simulink model "Wind_Turbine_Flexible_Blades"  (Simulink 7.9)
settings: Solver=ode15s  StartTime=0.0  StopTime=10  RelTol=1e-5
PreLoadFcn:
  | load ss_cantilever_pva.mat
  | warning('off','Simulink:SL_SaveWithParameterizedLinks_Warning');
PostLoadFcn:
  | loadMass = 20; %kg
InitFcn:
  | cantilever1=cantilever_aluminum;
  | load1.mass = 20 ; %kg
  | load1.inertia = eye(3) ; % assume point mass
  | load2=load1;
  | load2.angle = 35 * pi / 180;
undefined symbols (not defined in the file or in its folder): Flex_Blade
libraries: mblibv1 x21, Flex_Cantilever_Lib x3
Description:
  | Copyright 2011 MathWorks, Inc.
settings Model: Creator=smiller  LastModifiedBy=smiller
settings OptimizationCC: InitFltsAndDblsToZero=on
settings DebuggingCC: AlgebraicLoopMsg=none  ArtificialAlgebraicLoopMsg=none  SolverPrmCheckMsg=none  FcnCallInpInsideContextMsg=Use local settings  StrictBusMsg=Warning
settings GRTTargetCC: CombineOutputUpdateFcns=off  GRTInterface=on
settings SimMechanicsCC: VisSampleTime=0.1  AnimationDelay=0  LastVizWinPosition=[597 463 560 420]  CamPosition=[0.113022;0.0247231;-11.6929;]  CamTarget=[0.113022;0.0247231;-0;]  CamUpVector=[0;1;0;]  CamHeight=0.95142  VisBackgroundColor=[0.9;0.9;0.95;]  DefaultBodyColor=[1;0;0;]
settings ConfigurationSet: Description=SimMechanics 2G

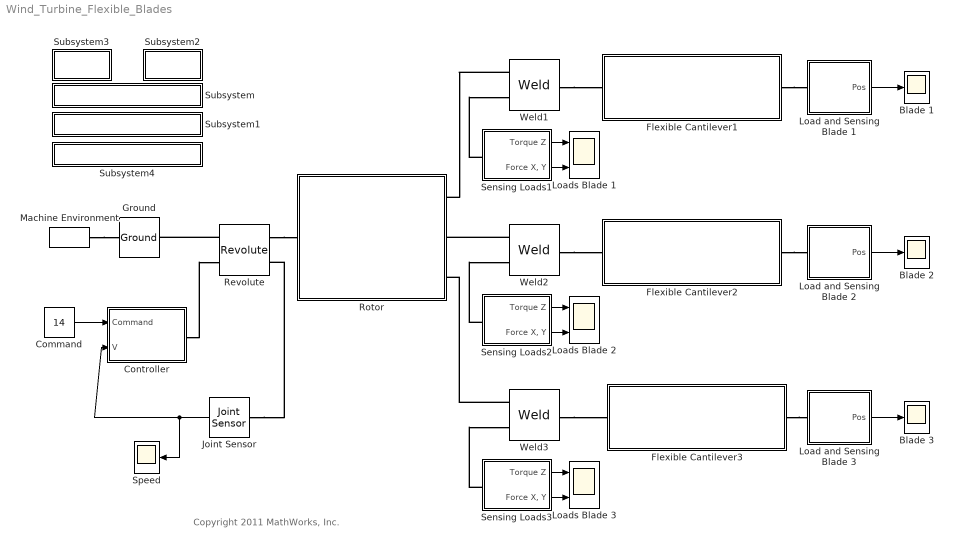
== system Wind_Turbine_Flexible_Blades ==
  note: Copyright 2011 MathWorks, Inc.
  Blade 1 : Scope
      settings: TimeRange=10  YMin=-0.6  YMax=0.6  SaveName=Flex_Beam_Tip_DATA1
  Blade 2 : Scope
      settings: TimeRange=10  YMin=-0.6  YMax=0.6  SaveName=Flex_Beam_Tip_DATA
  Blade 3 : Scope
      settings: TimeRange=10  YMin=-0.6  YMax=0.6  SaveName=Flex_Beam_Tip_DATA2
  Command : Constant  Value=14
  Controller : Subsystem
  Flexible Cantilever1 : Subsystem  BlockChoice=Lumped Parameter
      link override FEA Modes/Deflection due to flexibility/SIZED_INPUT_PORT: PortDimensions=3
      link override FEA Modes/Reaction Force on base (flexible body)/MSB_SIGNAL_BLOCK: Value=[0 0 0]
      link override Lumped Parameter/Beam1/Joint Sensor/MSB_SIGNAL_BLOCK: Value=0
      settings: AttributesFormatString=%<BlockChoice>  TemplateBlock=Flex_Cantilever_Lib/Flexible Cantilever  MemberBlocks=FEA Modes,Lumped Parameter
  Flexible Cantilever2 : Subsystem  BlockChoice=Lumped Parameter
      link override FEA Modes/Deflection due to flexibility/SIZED_INPUT_PORT: PortDimensions=3
      link override FEA Modes/Reaction Force on base (flexible body)/MSB_SIGNAL_BLOCK: Value=[0 0 0]
      link override Lumped Parameter/Beam1/Joint Sensor/MSB_SIGNAL_BLOCK: Value=0
      settings: AttributesFormatString=%<BlockChoice>  TemplateBlock=Flex_Cantilever_Lib/Flexible Cantilever  MemberBlocks=FEA Modes,Lumped Parameter
  Flexible Cantilever3 : Subsystem  BlockChoice=Lumped Parameter
      link override FEA Modes/Deflection due to flexibility/SIZED_INPUT_PORT: PortDimensions=3
      link override FEA Modes/Reaction Force on base (flexible body)/MSB_SIGNAL_BLOCK: Value=[0 0 0]
      link override Lumped Parameter/Beam1/Joint Sensor/MSB_SIGNAL_BLOCK: Value=0
      settings: AttributesFormatString=%<BlockChoice>  TemplateBlock=Flex_Cantilever_Lib/Flexible Cantilever  MemberBlocks=FEA Modes,Lumped Parameter
  Ground : mblibv1/Bodies/Ground  UpdateFromCAD=off  LeftPortType=env  RightPortType=workingframe  PhysicalDomain=Mechanical  DialogClass=GroundBlock  CoordPosition=[0 0 0]  CoordPositionUnits=m  StateVectorMgrId=-1  MachineId=[0 0]  ShowEnvPort=on
  Joint Sensor : mblibv1/Sensors &  Actuators/Joint Sensor  UpdateFromCAD=off  PhysicalDomain=Mechanical  PortType=blob  Muxed=off  Pose=off  Angle=off  AngleUnits=deg  ArcVelocity=on  ArcVelocityUnits=rpm  ArcAcceleration=off  ArcAccelerationUnits=deg/s^2  CoordPosition=on  CoordPositionUnits=m  Velocity=off  VelocityUnits=m/s  Acceleration=off  AccelerationUnits=m/s^2  Quaternion=on  QuaternionDT=off  QuaternionDDT=off  QuaternionUnits=off  OutputVector=[1]  ActiveIO=on  Width=1  DialogClass=MechanicalSensorBlock  Primitive=R1  Force=off  ForceUnits=N  Torque=off  TorqueUnits=N*m  ReferenceFrame=Absolute (World)  ReactionSensedSide=Base  ReactionReferenceFrame=Absolute (World)  ReactionForce=off  ReactionForceUnits=N  ReactionMoment=off  ReactionMomentUnits=N*m
  Load and Sensing Blade 1 : Subsystem
  Load and Sensing Blade 2 : Subsystem
  Load and Sensing Blade 3 : Subsystem
  Loads Blade 1 : Scope  NumInputPorts=2
      settings: TimeRange=10  YMin=-200~-400  YMax=200~200  SaveName=Flexible_Blade1_Load_DATA
  Loads Blade 2 : Scope  NumInputPorts=2
      settings: YMin=-400~-500  YMax=200~200
  Loads Blade 3 : Scope  NumInputPorts=2
      settings: YMin=-400~-500  YMax=200~200  SaveName=ScopeData3
  Machine Environment : mblibv1/Bodies/Machine Environment  Tag=Factory ground  PortType=env  PhysicalDomain=Mechanical  DialogTemplateClass=MECH.MachineEnvironment  SyncWhenCopied=off  Gravity=[0 -9.81 0]  GravityUnits=m/s^2  GravityAsSignal=off  Dimensionality=Auto-detect  AnalysisType=Forward dynamics  LinearAssemblyTolerance=1e-3  LinearAssemblyToleranceUnits=m  AngularAssemblyTolerance=1e-3  AngularAssemblyToleranceUnits=rad  ConstraintSolverType=Stabilizing  ConstraintRelTolerance=1e-4  ConstraintAbsTolerance=1e-4  UseRobustSingularityHandling=off  RedundancyAnalysisToleranceType=Automatically select tolerance  RedundancyAnalysisTolerance=1e-14  StatePerturbationType=Fixed  PerturbationSize=1e-5  VisualizeMachine=off  BodyVisualizationType=Use model default body geometries  BodyColorSelMode=Use model default  DefaultBodyColor=[1 0 0]
  Revolute : mblibv1/Joints/Revolute  LConnTagsString=__newl0|SA1  RConnTagsString=__newr0|SA1  UpdateFromCAD=off  NumSAPorts=2  CutJoint=off  MarkAsCut=off  Primitives=prismatic  PrimitiveProps=R1$World$[0 0 1]$revolute  DialogClass=JointBlock  R1Axis=[0 0 1]
  Rotor : Subsystem  mask(Disk){radius=0.325/8, width=0.06, mass=0.35, axis_pop=Z, x_angle=90, z_angle=0}
      mask prompts: radius "Radius (m)"; width "Length (m)"; mass "Mass (kg)"; axis_pop "Axis of Symmetry in ADJ Ref Frame"
      mask help: Represents a user-defined rigid body in the form of a cylinder. This dialog sets the mass, radius, length, and axis of symmetry. Axis of symmetry is defined by choosing the X, Y, or Z axis of the coordinate system attached to the ADJ port, which is parameterized using the ADJOINING option. The location of this body is parameterized to the coordinate system attached to the ADJ port.
      mask init:
      | if(strcmp(get_param(gcb,'axis_pop'),'X'))
      |     set_param(gcb,'x_angle','0');
      |     set_param(gcb,'z_angle','90');
      | elseif(strcmp(get_param(gcb,'axis_pop'),'Y'))
      |     set_param(gcb,'x_angle','0');
      |     set_param(gcb,'z_angle','0');
      | elseif(strcmp(get_param(gcb,'axis_pop'),'Z'))
      |     set_param(gcb,'x_angle','90');
      |     set_param(gcb,'z_angle','0');
      | end
      mask Help: Creates a cylindrical body
      mask StyleString: edit,edit,edit,popup(X|Y|Z),edit,edit
  Sensing Loads1 : Subsystem
  Sensing Loads2 : Subsystem
  Sensing Loads3 : Subsystem
  Speed : Scope
      settings: TimeRange=10  YMin=0  YMax=15  SaveName=Flexible_Blade_Rotor_Speed_DATA
  Subsystem : Subsystem
      settings: OpenFcn=Change_Flex_Body_To_FEA_Approach;
      mask Display: disp('Use FEA Modes')
  Subsystem1 : Subsystem
      settings: OpenFcn=Change_Flex_Body_To_Lumped_Parameter;
      mask Display: disp('Use Lumped Parameter')
  Subsystem2 : Subsystem
      settings: OpenFcn=|
      | Temp_ENVHa= get_param(find_system(gcs,'LookUnderMasks','all','FollowLinks','on','ClassName','Environment'),'handle');
      | 
      | set_param(Temp_ENVHa{1},'VisualizeMachine','off');
      | 
      | set_param(gcs,'VisDuringSimulation','off')
      | set_param(gcs,'VisOnUpdateDiagram','off')
      mask Display: disp('Vis Off')
  Subsystem3 : Subsystem
      settings: OpenFcn=|
      | Temp_ENVHa= get_param(find_system(gcs,'LookUnderMasks','all','FollowLinks','on','ClassName','Environment'),'handle');
      | 
      | set_param(Temp_ENVHa{1},'VisualizeMachine','on');
      | clear Temp_ENVHa;
      | set_param(gcs,'VisDuringSimulation','on')
      | set_param(gcs,'VisOnUpdateDiagram','on')
      mask Display: disp('Vis On')
  Subsystem4 : Subsystem
      settings: OpenFcn=Flexible_Blades_Slide_Prep;
      mask Display: disp('Show Methods')
  Weld1 : mblibv1/Joints/Weld  LConnTagsString=__newl0|SA1  RConnTagsString=__newr0  UpdateFromCAD=off  NumSAPorts=1  CutJoint=off  MarkAsCut=off  Primitives=weld  PrimitiveProps=W$World$[0 0 0]$weld  DialogClass=JointBlock  WAxis=[0 0 0]
  Weld2 : mblibv1/Joints/Weld  LConnTagsString=__newl0|SA1  RConnTagsString=__newr0  UpdateFromCAD=off  NumSAPorts=1  CutJoint=off  MarkAsCut=off  Primitives=weld  PrimitiveProps=W$World$[0 0 0]$weld  DialogClass=JointBlock  WAxis=[0 0 0]
  Weld3 : mblibv1/Joints/Weld  LConnTagsString=__newl0|SA1  RConnTagsString=__newr0  UpdateFromCAD=off  NumSAPorts=1  CutJoint=off  MarkAsCut=off  Primitives=weld  PrimitiveProps=W$World$[0 0 0]$weld  DialogClass=JointBlock  WAxis=[0 0 0]
  wires:
  Load and Sensing Blade 3/1(Pos) -> Blade 3/1
  Sensing Loads3/1(Torque Z) -> Loads Blade 3/1
  Load and Sensing Blade 1/1(Pos) -> Blade 1/1
  Sensing Loads1/1(Torque Z) -> Loads Blade 1/1
  Sensing Loads1/2("Force X, Y") -> Loads Blade 1/2
  Sensing Loads2/1(Torque Z) -> Loads Blade 2/1
  Sensing Loads2/2("Force X, Y") -> Loads Blade 2/2
  Joint Sensor/1 -> Controller/2(V), Speed/1
  Command/1 -> Controller/1(Command)
  Load and Sensing Blade 2/1(Pos) -> Blade 2/1
  Sensing Loads3/2("Force X, Y") -> Loads Blade 3/2
  connections:
  Sensing Loads1/LConn1 -- Weld1/LConn2
  Controller/RConn1 -- Revolute/LConn2
  Joint Sensor/LConn1 -- Revolute/RConn2
  Weld2/RConn1 -- Flexible Cantilever2/LConn1
  Weld2/LConn1 -- Rotor/RConn2
  Flexible Cantilever2/RConn1 -- Load and Sensing Blade 2/LConn1
  Sensing Loads2/LConn1 -- Weld2/LConn2
  Weld1/RConn1 -- Flexible Cantilever1/LConn1
  Revolute/LConn1 -- Ground/RConn1
  Flexible Cantilever1/RConn1 -- Load and Sensing Blade 1/LConn1
  Weld1/LConn1 -- Rotor/RConn1
  Revolute/RConn1 -- Rotor/LConn1
  Weld3/LConn1 -- Rotor/RConn3
  Sensing Loads3/LConn1 -- Weld3/LConn2
  Flexible Cantilever3/RConn1 -- Load and Sensing Blade 3/LConn1
  Weld3/RConn1 -- Flexible Cantilever3/LConn1
  Machine Environment/RConn1 -- Ground/LConn1

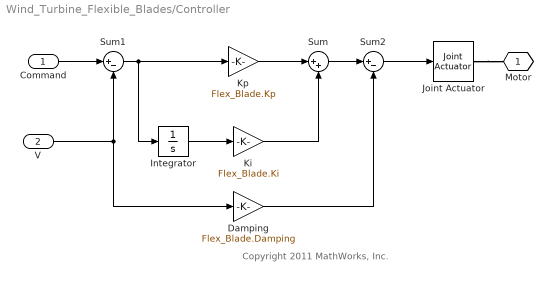
== system Wind_Turbine_Flexible_Blades/Controller ==
  note: Copyright 2011 MathWorks, Inc.
  Command : Inport
  V : Inport  Port=2
  Damping : Gain  Gain=Flex_Blade.Damping
  Integrator : Integrator
  Joint Actuator : mblibv1/Sensors &  Actuators/Joint Actuator  UpdateFromCAD=off  PhysicalDomain=Mechanical  PortType=blob  ActuationStyle=Force  AngleUnits=deg  ArcVelocityUnits=deg/s  ArcAccelerationUnits=deg/s^2  CoordPositionUnits=m  VelocityUnits=m/s  AccelerationUnits=m/s^2  ForceUnits=N  TorqueUnits=N*m  ActiveIO=on  Width=1  DialogClass=MechanicalActuatorBlock  Primitive=R1  ReferenceFrame=Absolute (World)
  Ki : Gain  Gain=Flex_Blade.Ki
  Kp : Gain  Gain=Flex_Blade.Kp
  Sum : Sum  Inputs=|++
  Sum1 : Sum  Inputs=|+-
  Sum2 : Sum  Inputs=|+-
  Motor : PMIOPort  Tag=PMCPort  Port=1  Side=Right
  wires:
  Sum1/1 -> Integrator/1, Kp/1
  Integrator/1 -> Ki/1
  Kp/1 -> Sum/1
  Ki/1 -> Sum/2
  Command/1 -> Sum1/1
  V/1 -> Sum1/2, Damping/1
  Sum/1 -> Sum2/1
  Sum2/1 -> Joint Actuator/1
  Damping/1 -> Sum2/2
  connections:
  Joint Actuator/RConn1 -- Motor/RConn1

== system Wind_Turbine_Flexible_Blades/Flexible Cantilever1 ==
  Lumped Parameter : Flex_Cantilever_Lib/Lumped Parameter  SystemSampleTime=-1
  Base : PMIOPort  Port=1  Side=Left
  Tip : PMIOPort  Port=2  Side=Right
  connections:
  Lumped Parameter/LConn1 -- Base/RConn1
  Lumped Parameter/RConn1 -- Tip/RConn1

== system Wind_Turbine_Flexible_Blades/Flexible Cantilever2 ==
  Lumped Parameter : Flex_Cantilever_Lib/Lumped Parameter  SystemSampleTime=-1
  Base : PMIOPort  Port=1  Side=Left
  Tip : PMIOPort  Port=2  Side=Right
  connections:
  Lumped Parameter/LConn1 -- Base/RConn1
  Lumped Parameter/RConn1 -- Tip/RConn1

== system Wind_Turbine_Flexible_Blades/Flexible Cantilever3 ==
  Lumped Parameter : Flex_Cantilever_Lib/Lumped Parameter  SystemSampleTime=-1
  Base : PMIOPort  Port=1  Side=Left
  Tip : PMIOPort  Port=2  Side=Right
  connections:
  Lumped Parameter/LConn1 -- Base/RConn1
  Lumped Parameter/RConn1 -- Tip/RConn1

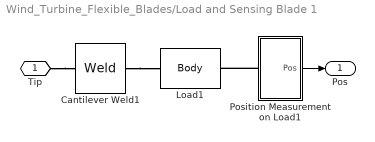
== system Wind_Turbine_Flexible_Blades/Load and Sensing Blade 1 ==
  Cantilever Weld1 : mblibv1/Joints/Weld  LConnTagsString=__newl0  RConnTagsString=__newr0  UpdateFromCAD=off  NumSAPorts=0  CutJoint=off  MarkAsCut=off  Primitives=weld  PrimitiveProps=W$WORLD$[0 0 0]$weld  DialogClass=JointBlock  WAxis=[0 0 0]
  Load1 : mblibv1/Bodies/Body  LConnTagsString=CS1  RConnTagsString=CS2  UpdateFromCAD=off  DialogClass=MechanicalBodyBlock  Mass=loadMass  MassUnits=kg  InertiaUnits=kg*m^2  Inertia=eye(3)  Shape=Cylinder  ShapeDims=[1 1]  ShapeUnits=m  ShapeUse=false  Density=1  DensityUnits=kg/m^3  DensityUse=false  GraphicsMode=1  BodyColorSelMode=MACHINE_DEFAULT  BodyColor=[0.5 0.5 0.5]  AttachedToCS=1  CG=Left$CG$[0 0 0]$CS1$CS1$m$[0 0 0]$Euler X-Y-Z$deg$CS1$false$none  WorkingFrames=Left$CS1$[0 0 0]$Adjoining$Adjoining$m$[0 0 0]$Euler X-Y-Z$deg$Adjoining$true$none#Right$CS2$[0 0 0]$CG$CG$m$[0 0 0]$Euler X-Y-Z$deg$CS1$true$none  CGPos=[0 0 0]  CGRot=[0 0 0]  CS0Pos=[]  CS0Rot=[]  CS1Pos=[0 0 0]  CS1Rot=[0 0 0]  CS2Pos=[0 0 0]  CS2Rot=[0 0 0]  CS3Pos=[]  CS3Rot=[]  CS4Pos=[]  CS4Rot=[]  CS5Pos=[]  CS5Rot=[]  CS6Pos=[]  CS6Rot=[]  CS7Pos=[]  CS7Rot=[]  CS8Pos=[]  CS8Rot=[]  CS9Pos=[]  CS9Rot=[]  CS10Pos=[]  CS10Rot=[]  CS11Pos=[]  CS11Rot=[]  CS12Pos=[]  CS12Rot=[]  CS13Pos=[]  CS13Rot=[]  CS14Pos=[]  CS14Rot=[]  CS15Pos=[]  CS15Rot=[]  CS16Pos=[]  CS16Rot=[]  CS17Pos=[]  CS17Rot=[]  CS18Pos=[]  CS18Rot=[]  CS19Pos=[]  CS19Rot=[]  CS20Pos=[]  CS20Rot=[]
  Position Measurement on Load1 : Subsystem
  Tip : PMIOPort  Port=1  Side=Left
  Pos : Outport
  wires:
  Position Measurement on Load1/1(Pos) -> Pos/1
  connections:
  Cantilever Weld1/LConn1 -- Load1/LConn1
  Position Measurement on Load1/LConn1 -- Load1/RConn1
  Tip/RConn1 -- Cantilever Weld1/RConn1

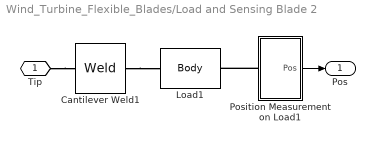
== system Wind_Turbine_Flexible_Blades/Load and Sensing Blade 2 ==
  Cantilever Weld1 : mblibv1/Joints/Weld  LConnTagsString=__newl0  RConnTagsString=__newr0  UpdateFromCAD=off  NumSAPorts=0  CutJoint=off  MarkAsCut=off  Primitives=weld  PrimitiveProps=W$WORLD$[0 0 0]$weld  DialogClass=JointBlock  WAxis=[0 0 0]
  Load1 : mblibv1/Bodies/Body  LConnTagsString=CS1  RConnTagsString=CS2  UpdateFromCAD=off  DialogClass=MechanicalBodyBlock  Mass=loadMass  MassUnits=kg  InertiaUnits=kg*m^2  Inertia=eye(3)  Shape=Cylinder  ShapeDims=[1 1]  ShapeUnits=m  ShapeUse=false  Density=1  DensityUnits=kg/m^3  DensityUse=false  GraphicsMode=1  BodyColorSelMode=MACHINE_DEFAULT  BodyColor=[0.5 0.5 0.5]  AttachedToCS=1  CG=Left$CG$[0 0 0]$CS1$CS1$m$[0 0 0]$Euler X-Y-Z$deg$CS1$false$none  WorkingFrames=Left$CS1$[0 0 0]$Adjoining$Adjoining$m$[0 0 0]$Euler X-Y-Z$deg$Adjoining$true$none#Right$CS2$[0 0 0]$CG$CG$m$[0 0 0]$Euler X-Y-Z$deg$CS1$true$none  CGPos=[0 0 0]  CGRot=[0 0 0]  CS0Pos=[]  CS0Rot=[]  CS1Pos=[0 0 0]  CS1Rot=[0 0 0]  CS2Pos=[0 0 0]  CS2Rot=[0 0 0]  CS3Pos=[]  CS3Rot=[]  CS4Pos=[]  CS4Rot=[]  CS5Pos=[]  CS5Rot=[]  CS6Pos=[]  CS6Rot=[]  CS7Pos=[]  CS7Rot=[]  CS8Pos=[]  CS8Rot=[]  CS9Pos=[]  CS9Rot=[]  CS10Pos=[]  CS10Rot=[]  CS11Pos=[]  CS11Rot=[]  CS12Pos=[]  CS12Rot=[]  CS13Pos=[]  CS13Rot=[]  CS14Pos=[]  CS14Rot=[]  CS15Pos=[]  CS15Rot=[]  CS16Pos=[]  CS16Rot=[]  CS17Pos=[]  CS17Rot=[]  CS18Pos=[]  CS18Rot=[]  CS19Pos=[]  CS19Rot=[]  CS20Pos=[]  CS20Rot=[]
  Position Measurement on Load1 : Subsystem
  Tip : PMIOPort  Port=1  Side=Left
  Pos : Outport
  wires:
  Position Measurement on Load1/1(Pos) -> Pos/1
  connections:
  Tip/RConn1 -- Cantilever Weld1/RConn1
  Position Measurement on Load1/LConn1 -- Load1/RConn1
  Cantilever Weld1/LConn1 -- Load1/LConn1

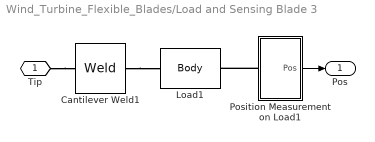
== system Wind_Turbine_Flexible_Blades/Load and Sensing Blade 3 ==
  Cantilever Weld1 : mblibv1/Joints/Weld  LConnTagsString=__newl0  RConnTagsString=__newr0  UpdateFromCAD=off  NumSAPorts=0  CutJoint=off  MarkAsCut=off  Primitives=weld  PrimitiveProps=W$WORLD$[0 0 0]$weld  DialogClass=JointBlock  WAxis=[0 0 0]
  Load1 : mblibv1/Bodies/Body  LConnTagsString=CS1  RConnTagsString=CS2  UpdateFromCAD=off  DialogClass=MechanicalBodyBlock  Mass=loadMass  MassUnits=kg  InertiaUnits=kg*m^2  Inertia=eye(3)  Shape=Cylinder  ShapeDims=[1 1]  ShapeUnits=m  ShapeUse=false  Density=1  DensityUnits=kg/m^3  DensityUse=false  GraphicsMode=1  BodyColorSelMode=MACHINE_DEFAULT  BodyColor=[0.5 0.5 0.5]  AttachedToCS=1  CG=Left$CG$[0 0 0]$CS1$CS1$m$[0 0 0]$Euler X-Y-Z$deg$CS1$false$none  WorkingFrames=Left$CS1$[0 0 0]$Adjoining$Adjoining$m$[0 0 0]$Euler X-Y-Z$deg$Adjoining$true$none#Right$CS2$[0 0 0]$CG$CG$m$[0 0 0]$Euler X-Y-Z$deg$CS1$true$none  CGPos=[0 0 0]  CGRot=[0 0 0]  CS0Pos=[]  CS0Rot=[]  CS1Pos=[0 0 0]  CS1Rot=[0 0 0]  CS2Pos=[0 0 0]  CS2Rot=[0 0 0]  CS3Pos=[]  CS3Rot=[]  CS4Pos=[]  CS4Rot=[]  CS5Pos=[]  CS5Rot=[]  CS6Pos=[]  CS6Rot=[]  CS7Pos=[]  CS7Rot=[]  CS8Pos=[]  CS8Rot=[]  CS9Pos=[]  CS9Rot=[]  CS10Pos=[]  CS10Rot=[]  CS11Pos=[]  CS11Rot=[]  CS12Pos=[]  CS12Rot=[]  CS13Pos=[]  CS13Rot=[]  CS14Pos=[]  CS14Rot=[]  CS15Pos=[]  CS15Rot=[]  CS16Pos=[]  CS16Rot=[]  CS17Pos=[]  CS17Rot=[]  CS18Pos=[]  CS18Rot=[]  CS19Pos=[]  CS19Rot=[]  CS20Pos=[]  CS20Rot=[]
  Position Measurement on Load1 : Subsystem
  Tip : PMIOPort  Port=1  Side=Left
  Pos : Outport
  wires:
  Position Measurement on Load1/1(Pos) -> Pos/1
  connections:
  Cantilever Weld1/LConn1 -- Load1/LConn1
  Position Measurement on Load1/LConn1 -- Load1/RConn1
  Tip/RConn1 -- Cantilever Weld1/RConn1

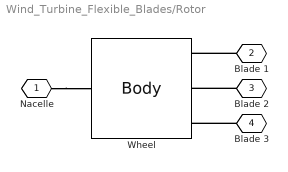
== system Wind_Turbine_Flexible_Blades/Rotor ==
  Wheel : mblibv1/Bodies/Body  LConnTagsString=CG  RConnTagsString=CS7|CS4|CS3  UpdateFromCAD=off  DialogClass=MechanicalBodyBlock  Mass=mass  MassUnits=kg  InertiaUnits=kg*m^2  Inertia=eye(3)  Shape=Cylinder  ShapeDims=[1 1]  ShapeUnits=m  ShapeUse=false  Density=1  DensityUnits=kg/m^3  DensityUse=false  GraphicsMode=1  BodyColorSelMode=MACHINE_DEFAULT  BodyColor=[0.5 0.5 0.5]  AttachedToCS=1  CG=Left$CG$[0 0 0]$ADJOINING$ADJOINING$m$[x_angle 0 z_angle]$Euler X-Y-Z$deg$ADJOINING$true$none  WorkingFrames=Right$CS1$[0 0 0]$CG$CG$m$[0 0 0]$Euler X-Y-Z$deg$CG$false$none#Right$CS5$[0 0 0]$CG$CG$m$[0 0 0]$Euler X-Y-Z$deg$CG$false$none#Right$CS7$[radius*cos(0*pi) 0 radius*sin(0*pi)]$CG$CG$m$[-90 0 0]$Euler X-Y-Z$deg$CG$true$none#Right$CS4$[radius*cos(0.666*pi) 0 radius*sin(0.666*pi)]$CG$CG$m$[-90 0 240]$Euler X-Y-Z$deg$CG$true$none#Right$CS3$[radius*cos(1.333*pi) 0 radius*sin(1.333*pi)]$CG$CG$m$[-90 0 120]$Euler X-Y-Z$deg$CG$true$none#Right$CS2$[radius*cos(0) -0.5*width radius*sin(0)]$CG$CG$m$[0 0 0]$Euler X-Y-Z$deg$CG$false$none#Right$CS17$[radius*cos(0) 0.5*width radius*sin(0)]$CG$CG$m$[0 0 0]$Euler X-Y-Z$deg$CG$false$none#Right$CS8$[radius*cos(0.2*pi) -0.5*width radius*sin(0.2*pi)]$CG$CG$m$[0 0 0]$Euler X-Y-Z$deg$CG$false$none#Right$CS18$[radius*cos(0.2*pi) 0.5*width radius*sin(0.2*pi)]$CG$CG$m$[0 0 0]$Euler X-Y-Z$deg$CG$false$none#Right$CS9$[radius*cos(0.4*pi) -0.5*width radius*sin(0.4*pi)]$CG$CG$m$[0 0 0]$Euler X-Y-Z$deg$CG$false$none#Right$CS19$[radius*cos(0.4*pi) 0.5*width radius*sin(0.4*pi)]$CG$CG$m$[0 0 0]$Euler X-Y-Z$deg$CG$false$none#Right$CS10$[radius*cos(0.6*pi) -0.5*width radius*sin(0.6*pi)]$CG$CG$m$[0 0 0]$Euler X-Y-Z$deg$CG$false$none#Right$CS20$[radius*cos(0.6*pi) 0.5*width radius*sin(0.6*pi)]$CG$CG$m$[0 0 0]$Euler X-Y-Z$deg$CG$false$none#Right$CS11$[radius*cos(0.8*pi) -0.5*width radius*sin(0.8*pi)]$CG$CG$m$[0 0 0]$Euler X-Y-Z$deg$CG$false$none#Right$CS21$[radius*cos(0.8*pi) 0.5*width radius*sin(0.8*pi)]$CG$CG$m$[0 0 0]$Euler X-Y-Z$deg$CG$false$none#Right$CS12$[radius*cos(1.0*pi) -0.5*width radius*sin(1.0*pi)]$CG$CG$m$[0 0 0]$Euler X-Y-Z$deg$CG$false$none#Right$CS22$[radius*cos(1.0*pi) 0.5*width radius*sin(1.0*pi)]$CG$CG$m$[0 0 0]$Euler X-Y-Z$deg$CG$false$none#Right$CS13$[radius*cos(1.2*pi) -0.5*width radius*sin(1.2*pi)]$CG$CG$m$[0 0 0]$Euler X-Y-Z$deg$CG$false$none#Right$CS23$[radius*cos(1.2*pi) 0.5*width radius*sin(1.2*pi)]$CG$CG$m$[0 0 0]$Euler X-Y-Z$deg$CG$false$none#Right$CS14$[radius*cos(1.4*pi) -0.5*width radius*sin(1.4*pi)]$CG$CG$m$[0 0 0]$Euler X-Y-Z$deg$CG$false$none#Right$CS24$[radius*cos(1.4*pi) 0.5*width radius*sin(1.4*pi)]$CG$CG$m$[0 0 0]$Euler X-Y-Z$deg$CG$false$none#Right$CS15$[radius*cos(1.6*pi) -0.5*width radius*sin(1.6*pi)]$CG$CG$m$[0 0 0]$Euler X-Y-Z$deg$CG$false$none#Right$CS25$[radius*cos(1.6*pi) 0.5*width radius*sin(1.6*pi)]$CG$CG$m$[0 0 0]$Euler X-Y-Z$deg$CG$false$none#Right$CS16$[radius*cos(1.8*pi) -0.5*width radius*sin(1.8*pi)]$CG$CG$m$[0 0 0]$Euler X-Y-Z$deg$CG$false$none#Right$CS26$[radius*cos(1.8*pi) 0.5*width radius*sin(1.8*pi)]$CG$CG$m$[0 0 0]$Euler X-Y-Z$deg$CG$false$none  CGPos=[0 0 0]  CGRot=[x_angle 0 z_angle]  CS0Pos=[]  CS0Rot=[]  CS1Pos=[0 0 0]  CS1Rot=[0 0 0]  CS2Pos=[radius*cos(0) -0.5*width radius*sin(0)]  CS2Rot=[0 0 0]  CS3Pos=[radius*cos(1.333*pi) 0 radius*sin(1.333*pi)]  CS3Rot=[-90 0 120]  CS4Pos=[radius*cos(0.666*pi) 0 radius*sin(0.666*pi)]  CS4Rot=[-90 0 240]  CS5Pos=[0 0 0]  CS5Rot=[0 0 0]  CS6Pos=[]  CS6Rot=[]  CS7Pos=[radius*cos(0*pi) 0 radius*sin(0*pi)]  CS7Rot=[-90 0 0]  CS8Pos=[radius*cos(0.2*pi) -0.5*width radius*sin(0.2*pi)]  CS8Rot=[0 0 0]  CS9Pos=[radius*cos(0.4*pi) -0.5*width radius*sin(0.4*pi)]  CS9Rot=[0 0 0]  CS10Pos=[radius*cos(0.6*pi) -0.5*width radius*sin(0.6*pi)]  CS10Rot=[0 0 0]  CS11Pos=[radius*cos(0.8*pi) -0.5*width radius*sin(0.8*pi)]  CS11Rot=[0 0 0]  CS12Pos=[radius*cos(1.0*pi) -0.5*width radius*sin(1.0*pi)]  CS12Rot=[0 0 0]  CS13Pos=[radius*cos(1.2*pi) -0.5*width radius*sin(1.2*pi)]  CS13Rot=[0 0 0]  CS14Pos=[radius*cos(1.4*pi) -0.5*width radius*sin(1.4*pi)]  CS14Rot=[0 0 0]  CS15Pos=[radius*cos(1.6*pi) -0.5*width radius*sin(1.6*pi)]  CS15Rot=[0 0 0]  CS16Pos=[radius*cos(1.8*pi) -0.5*width radius*sin(1.8*pi)]  CS16Rot=[0 0 0]  CS17Pos=[radius*cos(0) 0.5*width radius*sin(0)]  CS17Rot=[0 0 0]  CS18Pos=[radius*cos(0.2*pi) 0.5*width radius*sin(0.2*pi)]  CS18Rot=[0 0 0]  CS19Pos=[radius*cos(0.4*pi) 0.5*width radius*sin(0.4*pi)]  CS19Rot=[0 0 0]  CS20Pos=[radius*cos(0.6*pi) 0.5*width radius*sin(0.6*pi)]  CS20Rot=[0 0 0]
  " Nacelle" : PMIOPort  Tag=PMCPort  Port=1  Side=Left
  Blade 1 : PMIOPort  Tag=PMCPort  Port=2  Side=Right
  Blade 2 : PMIOPort  Tag=PMCPort  Port=3  Side=Right
  Blade 3 : PMIOPort  Tag=PMCPort  Port=4  Side=Right
  connections:
  " Nacelle"/RConn1 -- Wheel/LConn1
  Blade 1/RConn1 -- Wheel/RConn1
  Blade 2/RConn1 -- Wheel/RConn2
  Blade 3/RConn1 -- Wheel/RConn3

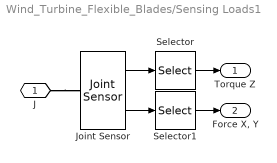
== system Wind_Turbine_Flexible_Blades/Sensing Loads1 ==
  Joint Sensor : mblibv1/Sensors &  Actuators/Joint Sensor  UpdateFromCAD=off  PhysicalDomain=Mechanical  PortType=blob  Muxed=off  Pose=off  Angle=on  AngleUnits=deg  ArcVelocity=off  ArcVelocityUnits=deg/s  ArcAcceleration=off  ArcAccelerationUnits=deg/s^2  CoordPosition=on  CoordPositionUnits=m  Velocity=off  VelocityUnits=m/s  Acceleration=off  AccelerationUnits=m/s^2  Quaternion=on  QuaternionDT=off  QuaternionDDT=off  QuaternionUnits=off  OutputVector=[1]  ActiveIO=on  Width=6  DialogClass=MechanicalSensorBlock  Primitive=W  Force=off  ForceUnits=N  Torque=off  TorqueUnits=N*m  ReferenceFrame=Absolute (World)  ReactionSensedSide=Base  ReactionReferenceFrame=Absolute (World)  ReactionForce=on  ReactionForceUnits=N  ReactionMoment=on  ReactionMomentUnits=N*m
  Selector : Selector  InputPortWidth=3  IndexOptions=Index vector (dialog)  Indices=[3]  OutputSizes=1
  Selector1 : Selector  InputPortWidth=3  IndexOptions=Index vector (dialog)  Indices=[1 2]  OutputSizes=1
  J : PMIOPort  Port=1  Side=Left
  Torque Z : Outport
  "Force X, Y" : Outport  Port=2
  wires:
  Selector1/1 -> "Force X, Y"/1
  Selector/1 -> Torque Z/1
  Joint Sensor/2 -> Selector1/1
  Joint Sensor/1 -> Selector/1
  connections:
  J/RConn1 -- Joint Sensor/LConn1

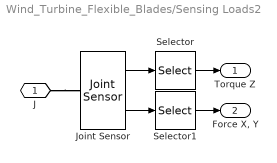
== system Wind_Turbine_Flexible_Blades/Sensing Loads2 ==
  Joint Sensor : mblibv1/Sensors &  Actuators/Joint Sensor  UpdateFromCAD=off  PhysicalDomain=Mechanical  PortType=blob  Muxed=off  Pose=off  Angle=on  AngleUnits=deg  ArcVelocity=off  ArcVelocityUnits=deg/s  ArcAcceleration=off  ArcAccelerationUnits=deg/s^2  CoordPosition=on  CoordPositionUnits=m  Velocity=off  VelocityUnits=m/s  Acceleration=off  AccelerationUnits=m/s^2  Quaternion=on  QuaternionDT=off  QuaternionDDT=off  QuaternionUnits=off  OutputVector=[1]  ActiveIO=on  Width=6  DialogClass=MechanicalSensorBlock  Primitive=W  Force=off  ForceUnits=N  Torque=off  TorqueUnits=N*m  ReferenceFrame=Absolute (World)  ReactionSensedSide=Base  ReactionReferenceFrame=Absolute (World)  ReactionForce=on  ReactionForceUnits=N  ReactionMoment=on  ReactionMomentUnits=N*m
  Selector : Selector  InputPortWidth=3  IndexOptions=Index vector (dialog)  Indices=[3]  OutputSizes=1
  Selector1 : Selector  InputPortWidth=3  IndexOptions=Index vector (dialog)  Indices=[1 2]  OutputSizes=1
  J : PMIOPort  Port=1  Side=Left
  Torque Z : Outport
  "Force X, Y" : Outport  Port=2
  wires:
  Joint Sensor/1 -> Selector/1
  Joint Sensor/2 -> Selector1/1
  Selector/1 -> Torque Z/1
  Selector1/1 -> "Force X, Y"/1
  connections:
  J/RConn1 -- Joint Sensor/LConn1

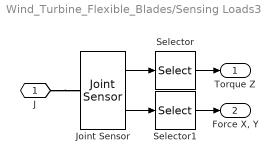
== system Wind_Turbine_Flexible_Blades/Sensing Loads3 ==
  Joint Sensor : mblibv1/Sensors &  Actuators/Joint Sensor  UpdateFromCAD=off  PhysicalDomain=Mechanical  PortType=blob  Muxed=off  Pose=off  Angle=on  AngleUnits=deg  ArcVelocity=off  ArcVelocityUnits=deg/s  ArcAcceleration=off  ArcAccelerationUnits=deg/s^2  CoordPosition=on  CoordPositionUnits=m  Velocity=off  VelocityUnits=m/s  Acceleration=off  AccelerationUnits=m/s^2  Quaternion=on  QuaternionDT=off  QuaternionDDT=off  QuaternionUnits=off  OutputVector=[1]  ActiveIO=on  Width=6  DialogClass=MechanicalSensorBlock  Primitive=W  Force=off  ForceUnits=N  Torque=off  TorqueUnits=N*m  ReferenceFrame=Absolute (World)  ReactionSensedSide=Base  ReactionReferenceFrame=Absolute (World)  ReactionForce=on  ReactionForceUnits=N  ReactionMoment=on  ReactionMomentUnits=N*m
  Selector : Selector  InputPortWidth=3  IndexOptions=Index vector (dialog)  Indices=[3]  OutputSizes=1
  Selector1 : Selector  InputPortWidth=3  IndexOptions=Index vector (dialog)  Indices=[1 2]  OutputSizes=1
  J : PMIOPort  Port=1  Side=Left
  Torque Z : Outport
  "Force X, Y" : Outport  Port=2
  wires:
  Selector1/1 -> "Force X, Y"/1
  Selector/1 -> Torque Z/1
  Joint Sensor/2 -> Selector1/1
  Joint Sensor/1 -> Selector/1
  connections:
  J/RConn1 -- Joint Sensor/LConn1

== system Wind_Turbine_Flexible_Blades/Subsystem ==

== system Wind_Turbine_Flexible_Blades/Subsystem1 ==

== system Wind_Turbine_Flexible_Blades/Subsystem2 ==

== system Wind_Turbine_Flexible_Blades/Subsystem3 ==

== system Wind_Turbine_Flexible_Blades/Subsystem4 ==

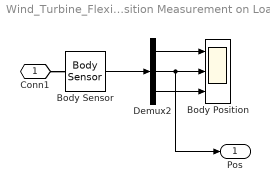
== system Wind_Turbine_Flexible_Blades/Load and Sensing Blade 1/Position Measurement on Load1 ==
  Body Position : Scope  NumInputPorts=3
      settings: TimeRange=0.3  YMin=0.599997~-0.0065~-1  YMax=0.6~0~1  SaveName=ScopeData2
  Body Sensor : mblibv1/Sensors &  Actuators/Body Sensor  UpdateFromCAD=off  PhysicalDomain=Mechanical  PortType=blob  Muxed=on  Pose=off  Angle=on  AngleUnits=deg  ArcVelocity=off  ArcVelocityUnits=deg/s  ArcAcceleration=off  ArcAccelerationUnits=deg/s^2  CoordPosition=on  CoordPositionUnits=m  Velocity=off  VelocityUnits=m/s  Acceleration=off  AccelerationUnits=m/s^2  Quaternion=on  QuaternionDT=off  QuaternionDDT=off  QuaternionUnits=off  OutputVector=[1]  ActiveIO=on  Width=3  DialogClass=MechanicalSensorBlock  ReferenceFrame=Absolute (World)
  Demux2 : Demux  Outputs=3
  Conn1 : PMIOPort  Port=1  Side=Left
  Pos : Outport
  wires:
  Demux2/3 -> Body Position/3
  Demux2/2 -> Body Position/2, Pos/1
  Demux2/1 -> Body Position/1
  Body Sensor/1 -> Demux2/1
  connections:
  Conn1/RConn1 -- Body Sensor/LConn1

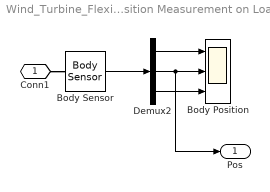
== system Wind_Turbine_Flexible_Blades/Load and Sensing Blade 2/Position Measurement on Load1 ==
  Body Position : Scope  NumInputPorts=3
      settings: TimeRange=0.3  YMin=0.599997~-0.0065~-1  YMax=0.6~0~1  SaveName=ScopeData2
  Body Sensor : mblibv1/Sensors &  Actuators/Body Sensor  UpdateFromCAD=off  PhysicalDomain=Mechanical  PortType=blob  Muxed=on  Pose=off  Angle=on  AngleUnits=deg  ArcVelocity=off  ArcVelocityUnits=deg/s  ArcAcceleration=off  ArcAccelerationUnits=deg/s^2  CoordPosition=on  CoordPositionUnits=m  Velocity=off  VelocityUnits=m/s  Acceleration=off  AccelerationUnits=m/s^2  Quaternion=on  QuaternionDT=off  QuaternionDDT=off  QuaternionUnits=off  OutputVector=[1]  ActiveIO=on  Width=3  DialogClass=MechanicalSensorBlock  ReferenceFrame=Absolute (World)
  Demux2 : Demux  Outputs=3
  Conn1 : PMIOPort  Port=1  Side=Left
  Pos : Outport
  wires:
  Body Sensor/1 -> Demux2/1
  Demux2/1 -> Body Position/1
  Demux2/2 -> Pos/1, Body Position/2
  Demux2/3 -> Body Position/3
  connections:
  Conn1/RConn1 -- Body Sensor/LConn1

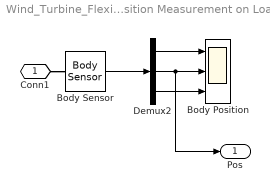
== system Wind_Turbine_Flexible_Blades/Load and Sensing Blade 3/Position Measurement on Load1 ==
  Body Position : Scope  NumInputPorts=3
      settings: TimeRange=0.3  YMin=0.599997~-0.0065~-1  YMax=0.6~0~1  SaveName=ScopeData2
  Body Sensor : mblibv1/Sensors &  Actuators/Body Sensor  UpdateFromCAD=off  PhysicalDomain=Mechanical  PortType=blob  Muxed=on  Pose=off  Angle=on  AngleUnits=deg  ArcVelocity=off  ArcVelocityUnits=deg/s  ArcAcceleration=off  ArcAccelerationUnits=deg/s^2  CoordPosition=on  CoordPositionUnits=m  Velocity=off  VelocityUnits=m/s  Acceleration=off  AccelerationUnits=m/s^2  Quaternion=on  QuaternionDT=off  QuaternionDDT=off  QuaternionUnits=off  OutputVector=[1]  ActiveIO=on  Width=3  DialogClass=MechanicalSensorBlock  ReferenceFrame=Absolute (World)
  Demux2 : Demux  Outputs=3
  Conn1 : PMIOPort  Port=1  Side=Left
  Pos : Outport
  wires:
  Demux2/3 -> Body Position/3
  Demux2/2 -> Body Position/2, Pos/1
  Demux2/1 -> Body Position/1
  Body Sensor/1 -> Demux2/1
  connections:
  Conn1/RConn1 -- Body Sensor/LConn1
